simulink model "PendulumInverseSIMU_L"  (Simulink 10.0)
settings: Solver=ode45  StartTime=ti  StopTime=tf  FixedStep=0.001  RelTol=1e-3  EnableMultiTasking=on
undefined symbols (not defined in the file): A_Obs, B_Obs, C_Obs, D_Obs, g, Initial, J, K, l, m, Mcart, Noise, Observer
libraries: simulink x1
settings Model: Creator=huojiaxi  LastModifiedBy=huojiaxi  ExtModeTrigMode=oneshot  ExtModeArmWhenConnect=off
settings DataIOCC: SignalLoggingSaveFormat=ModelDataLogs
settings OptimizationCC: BooleanDataType=off  LifeSpan=auto
settings DebuggingCC: SaveWithParameterizedLinksMsg=none  SignalResolutionControl=TryResolveAllWithWarning  MultiTaskDSMMsg=warning  MultiTaskCondExecSysMsg=none  SFUnexpectedBacktrackingDiag=error  SFNoUnconditionalDefaultTransitionDiag=error  SFExecutionAtInitializationDiag=warning  ArithmeticOperatorsInVariantConditions=error
settings HardwareCC: ProdBitPerPointer=64  ProdBitPerSizeT=64  ProdBitPerPtrDiffT=64  ProdLargestAtomicFloat=Float  ProdIntDivRoundTo=Zero  ProdEndianess=LittleEndian  ProdWordSize=64  ProdHWDeviceType=Intel->x86-64 (Windows64)  TargetUnknown=on
settings SFSimCC: SimUseLocalCustomCode=on  CustomCodeUndefinedFunction=FilterOut
settings RTWCC: RTWUseLocalCustomCode=on
settings CodeAppCC: StateflowObjectComments=off
settings GRTTargetCC: TargetLangStandard=C99 (ISO)
settings ConfigComp: CovSaveCumulativeToWorkspaceVar=off  CovSaveSingleToWorkspaceVar=off

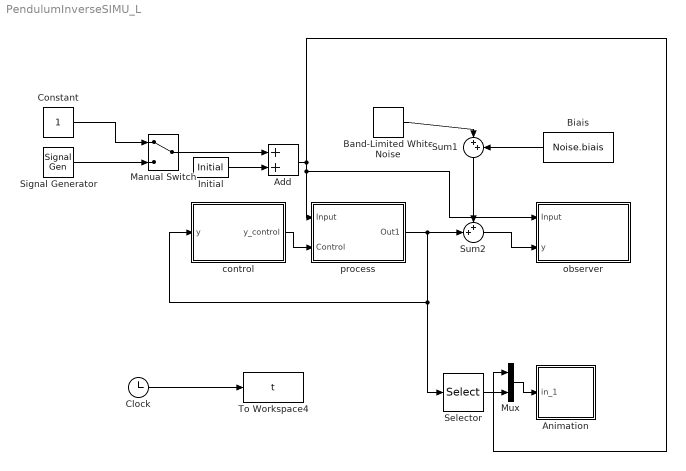
== system PendulumInverseSIMU_L ==
  Add : Sum
  Animation : Subsystem  mask(Pendulum plot){RefBlock=Initial}
      mask prompts: RefBlock "DC reference signal block name:"
      mask help: Pendulum plot
      mask Help: Pendulum animation function using Handle graphics.
      mask Display: plot([-10 10],[0 0],[-2 -2 2 2],[0 1 1 0],[0 3],[1 5])
  Band-Limited White Noise : simulink/Sources/Band-Limited White Noise  Cov=Noise.power  Ts=Noise.sampling  seed=Noise.seed
  Biais : Constant  Value=Noise.biais
  Clock : Clock
  Constant : Constant
  Initial : Constant  Value=Initial
  Manual Switch : ManualSwitch
  Mux : Mux  Inputs=2
  Selector : Selector  InputPortWidth=4  IndexOptions=Index vector (dialog)  Indices=[3 1]  OutputSizes=1
  Signal Generator : SignalGenerator  Units=rad/sec
  Sum1 : Sum  Inputs=|++
  Sum2 : Sum  Inputs=++|
  To Workspace4 : ToWorkspace  VariableName=t  SampleTime=-1
  control : Subsystem
  observer : Subsystem
  process : Subsystem
  wires:
  control/1(y_control) -> process/2(Control)
  Clock/1 -> To Workspace4/1
  process/1(Out1) -> Sum2/2, Selector/1, control/1(y)
  Manual Switch/1 -> Add/1
  Band-Limited White Noise/1 -> Sum1/1
  Sum1/1 -> Sum2/1
  Biais/1 -> Sum1/2
  Sum2/1 -> observer/2(y)
  Constant/1 -> Manual Switch/1
  Signal Generator/1 -> Manual Switch/2
  Selector/1 -> Mux/2
  Mux/1 -> Animation/1(in_1)
  Initial/1 -> Add/2
  Add/1 -> process/1(Input), observer/1(Input), Mux/1

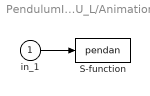
== system PendulumInverseSIMU_L/Animation ==
  in_1 : Inport
  S-function : S-Function  FunctionName=pendan  Parameters=RefBlock  SFunctionDeploymentMode=off  EnableBusSupport=off
      settings: DeleteFcn=pendan([],[],[],'DeleteBlock');
  wires:
  in_1/1 -> S-function/1

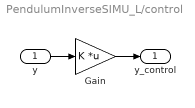
== system PendulumInverseSIMU_L/control ==
  y : Inport
  Gain : Gain  Gain=K  Multiplication=Matrix(K*u) (u vector)
  y_control : Outport
  wires:
  y/1 -> Gain/1
  Gain/1 -> y_control/1

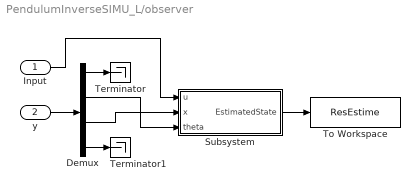
== system PendulumInverseSIMU_L/observer ==
  Input : Inport
  y : Inport  Port=2
  Demux : Demux
  Subsystem : Subsystem
  Terminator : Terminator
  Terminator1 : Terminator
  To Workspace : ToWorkspace  VariableName=ResEstime  SampleTime=-1
  wires:
  y/1 -> Demux/1
  Demux/4 -> Terminator1/1
  Demux/1 -> Terminator/1
  Demux/3 -> Subsystem/2("x ")
  Demux/2 -> Subsystem/3(theta)
  Input/1 -> Subsystem/1(u)
  Subsystem/1(EstimatedState) -> To Workspace/1

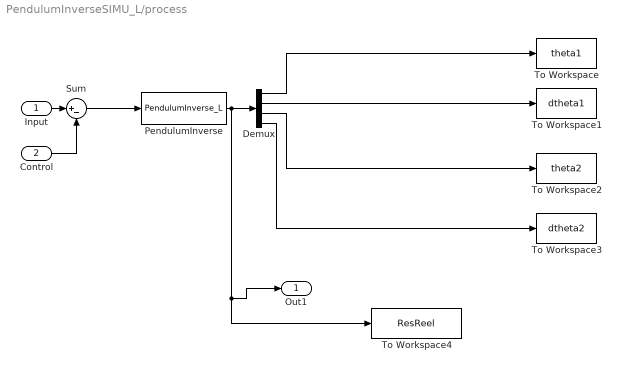
== system PendulumInverseSIMU_L/process ==
  Input : Inport
  Control : Inport  Port=2
  Demux : Demux
  PendulumInverse : S-Function  FunctionName=PendulumInverse_L  Parameters=Mcart,m,l,g,J  SFunctionDeploymentMode=off  EnableBusSupport=off
  Sum : Sum  Inputs=|+-
  To Workspace : ToWorkspace  VariableName=theta1  SampleTime=-1
  To Workspace1 : ToWorkspace  VariableName=dtheta1  SampleTime=-1
  To Workspace2 : ToWorkspace  VariableName=theta2  SampleTime=-1
  To Workspace3 : ToWorkspace  VariableName=dtheta2  SampleTime=-1
  To Workspace4 : ToWorkspace  VariableName=ResReel  SampleTime=-1
  Out1 : Outport
  wires:
  PendulumInverse/1 -> Demux/1, To Workspace4/1, Out1/1
  Demux/3 -> To Workspace2/1
  Demux/2 -> To Workspace1/1
  Demux/1 -> To Workspace/1
  Demux/4 -> To Workspace3/1
  Input/1 -> Sum/1
  Control/1 -> Sum/2
  Sum/1 -> PendulumInverse/1

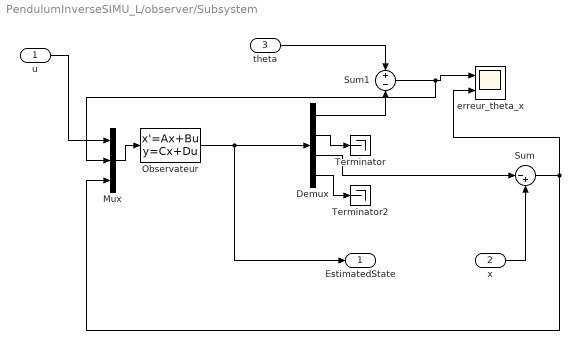
== system PendulumInverseSIMU_L/observer/Subsystem ==
  u : Inport
  "x " : Inport  Port=2
  theta : Inport  Port=3
  Demux : Demux
  Mux : Mux  Inputs=3
  Observateur : StateSpace  A=A_Obs  B=B_Obs  C=C_Obs  D=D_Obs  InitialCondition=Observer.IC
  Sum : Sum  Inputs=|-+
  Sum1 : Sum  Inputs=+-
  Terminator : Terminator
  Terminator2 : Terminator
  erreur_theta_x : Scope  NumInputPorts=2
  EstimatedState : Outport  VectorParamsAs1DForOutWhenUnconnected=off
  wires:
  Demux/3 -> Sum/1
  Demux/2 -> Terminator/1
  Mux/1 -> Observateur/1
  theta/1 -> Sum1/1
  Demux/1 -> Sum1/2
  u/1 -> Mux/1
  Sum1/1 -> Mux/2, erreur_theta_x/1
  Observateur/1 -> EstimatedState/1, Demux/1
  Demux/4 -> Terminator2/1
  "x "/1 -> Sum/2
  Sum/1 -> erreur_theta_x/2, Mux/3
